simulink model "TWO_DOF_PID"  (R2023b)
settings: Solver=VariableStepAuto  StartTime=0.0  StopTime=10.0  RelTol=1e-3
undefined symbols (not defined in the file): beta_yaw, cneg, cpos, Dt, fd, force_coef, fs, I_omega, Jy, kTn1, kTn2, kTp1, kTp2, P_omega, parameters
libraries: slpidlib x3
settings Model: Creator=franc  LastModifiedBy=franc

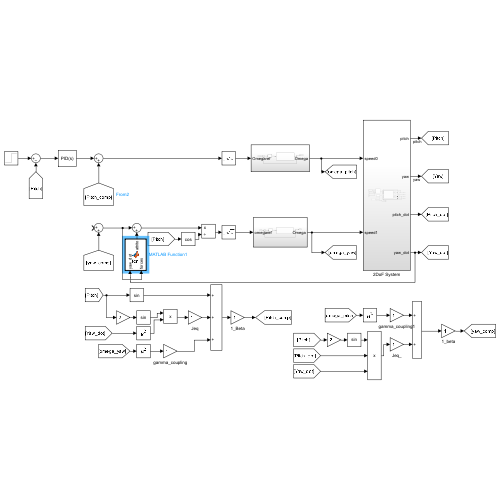
[thumbnail: Simulink's stored preview of the top-level diagram]
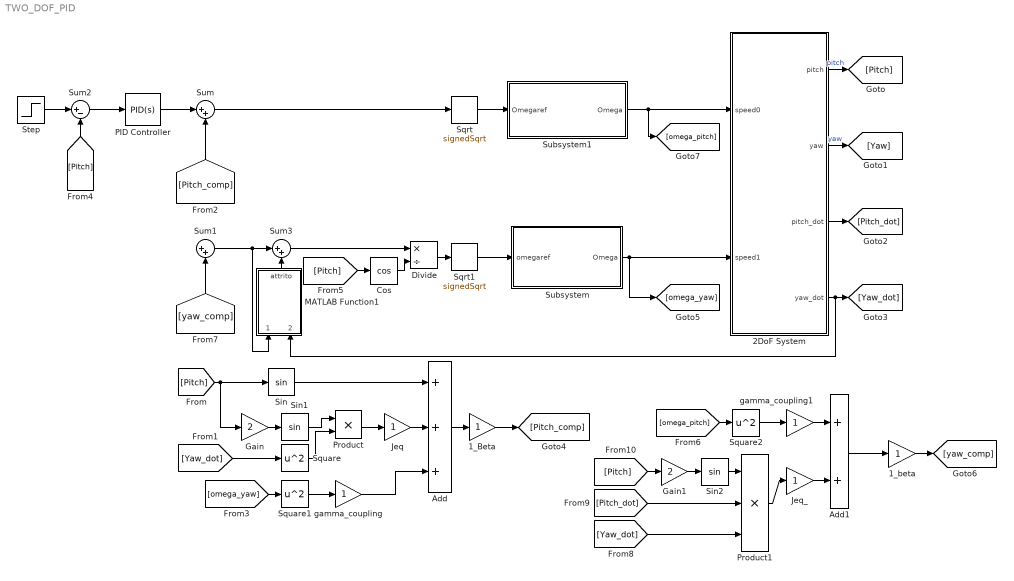
== system TWO_DOF_PID ==
  1_Beta : Gain
  1_beta : Gain
  2DoF System : Subsystem
  Add : Sum  Inputs=+++
  Add1 : Sum
  Cos : Trigonometry  Operator=cos
  Divide : Product  Inputs=*/
  Gain : Gain  Gain=2
  Gain1 : Gain  Gain=2
  Jeq : Gain
  Jeq_ : Gain
  MATLAB Function1 : MATLAB Function  TreatAsAtomicUnit=on
  PID Controller : slpidlib/PID Controller  Controller=PID  Form=Parallel  TimeDomain=Continuous-time  UseExternalTs=off  SampleTime=-1  IntegratorMethod=Forward Euler  FilterMethod=Forward Euler  ControllerParametersSource=internal  P=1  I=1  UseKiTs=off  D=0  N=100  UseFilter=on  TunerSelectOption=Transfer Function Based (PID Tuner App)  InitialConditionSource=internal  InitialConditionForIntegrator=0  InitialConditionForFilter=0  DifferentiatorICPrevScaledInput=0  ExternalReset=none  TrackingMode=off  Kt=1  LimitOutput=off  SatLimitsSource=internal  UpperSaturationLimit=inf  LowerSaturationLimit=-inf  LinearizeAsGain=on  AntiWindupMode=none  Kb=1  LimitIntegrator=off  UpperIntegratorSaturationLimit=inf  LowerIntegratorSaturationLimit=-inf  POutMin=[]  POutMax=[]  IOutMin=[]  IOutMax=[]  DOutMin=[]  DOutMax=[]  NOutMin=[]  NOutMax=[]  SumOutMin=[]  SumOutMax=[]  SaturationOutMin=[]  SaturationOutMax=[]  PParamMin=[]  PParamMax=[]  IParamMin=[]  IParamMax=[]  DParamMin=[]  DParamMax=[]  NParamMin=[]  NParamMax=[]  KbParamMin=[]  KbParamMax=[]  KtParamMin=[]  KtParamMax=[]  KbOutMin=[]  KbOutMax=[]  KtOutMin=[]  KtOutMax=[]  IntegratorOutMin=[]  IntegratorOutMax=[]  FilterOutMin=[]  FilterOutMax=[]  SumI1OutMin=[]  SumI1OutMax=[]  SumI2OutMin=[]  SumI2OutMax=[]  SumI3OutMin=[]  SumI3OutMax=[]  SumI4OutMin=[]  SumI4OutMax=[]  SumDOutMin=[]  SumDOutMax=[]  DifferentiatorOutMin=[]  DifferentiatorOutMax=[]  FilterDiffOutCoefMin=[]  FilterDiffOutCoefMax=[]  ReciprocalOutMin=[]  ReciprocalOutMax=[]  SumDenOutMin=[]  SumDenOutMax=[]  SumNumOutMin=[]  SumNumOutMax=[]  DivideOutMin=[]  DivideOutMax=[]  UdiffTsProdOutMin=[]  UdiffTsProdOutMax=[]  NTsProdOutMin=[]  NTsProdOutMax=[]  UintegralTsProdOutMin=[]  UintegralTsProdOutMax=[]  UngainTsProdOutMin=[]  UngainTsProdOutMax=[]  ClampingZeroOutDataTypeStr=Inherit: Inherit via back propagation  ClampingZeroOutMin=[]  ClampingZeroOutMax=[]  FilterDenConstantOutDataTypeStr=Inherit: Inherit via back propagation  FilterDenConstantOutMin=[]  FilterDenConstantOutMax=[]  PCopyOutDataTypeStr=Inherit: Inherit via back propagation  PCopyOutMin=[]  PCopyOutMax=[]  NCopyOutDataTypeStr=Inherit: Inherit via back propagation  NCopyOutMin=[]  NCopyOutMax=[]  IntegratorContinuousStateAttributes=''  IntegratorStateMustResolveToSignalObject=off  IntegratorRTWStateStorageClass=Auto  FilterContinuousStateAttributes=''  FilterStateMustResolveToSignalObject=off  FilterRTWStateStorageClass=Auto  ParallelPVariant=InternalParameters  IdealPVariant=Disabled  IVariant=InternalParameters  DVariant=InternalParameters  IntegratorVariant=Continuous  SatVariant=Disabled  AWVariant=Passthrough  PCopyVariant=Disabled  TRVariant=Disabled  FdbkBlocksVariant=Forward  IdealPFdbkVariant=Disabled  SatFdbkVariant=Disabled  DerivativeFilterVariant=ContFilter  NVariant=InternalParameters  NCopyVariant=Disabled  FilterICVariant=InternalICsFilter  IntegratorICVariant=InternalICs  ExternalResetVariant=Disabled  TRSumVariant=Passthrough  SumFdbkVariant=Disabled  SumVariant=Sum_PID  TsampFilterVariant=InternalTs  TsampNgainVariant=Passthrough  TsampIntegralVariant=Passthrough  ExternalSaturationOutDataTypeStr=Inherit: Same as second input
  Product : Product
  Product1 : Product  Inputs=3
  Sin : Trigonometry
  Sin1 : Trigonometry
  Sin2 : Trigonometry
  Sqrt : Sqrt  Operator=signedSqrt
  Sqrt1 : Sqrt  Operator=signedSqrt
  Square : Math  Operator=square
  Square1 : Math  Operator=square
  Square2 : Math  Operator=square
  Step : Step  After=30*pi/180  SampleTime=0
  Subsystem : Subsystem
  Subsystem1 : Subsystem
  Sum : Sum  Inputs=|++
  Sum1 : Sum  Inputs=|++
  Sum2 : Sum  Inputs=|+-
  Sum3 : Sum  Inputs=|++
  gamma_coupling : Gain
  gamma_coupling1 : Gain
  wires:
  Subsystem/1(Omega) -> [omega_yaw], 2DoF System/2(speed1)
  Subsystem1/1(Omega) -> [omega_pitch], 2DoF System/1(speed0)
  Sqrt/1 -> Subsystem1/1(Omegaref)
  Sqrt1/1 -> Subsystem/1(omegaref)
  Sum3/1 -> Divide/1
  Sum/1 -> Sqrt/1
  2DoF System/1(pitch) -> [Pitch]  "pitch"
  2DoF System/2(yaw) -> [Yaw]  "yaw"
  2DoF System/3(pitch_dot) -> [Pitch_dot]
  2DoF System/4(yaw_dot) -> MATLAB Function1/2(yaw_dot), [Yaw_dot]
  [Pitch] -> Gain/1, Sin/1
  Sin/1 -> Add/1
  Gain/1 -> Sin1/1
  Sin1/1 -> Product/1
  Jeq/1 -> Add/2
  [Yaw_dot] -> Square/1
  Product/1 -> Jeq/1
  Add/1 -> 1_Beta/1
  [Pitch_comp] -> Sum/2
  Square/1 -> Product/2
  [omega_yaw] -> Square1/1
  Square1/1 -> gamma_coupling/1
  gamma_coupling/1 -> Add/3
  PID Controller/1 -> Sum/1
  Sum2/1 -> PID Controller/1
  [Pitch] -> Sum2/2
  1_Beta/1 -> [Pitch_comp]
  Step/1 -> Sum2/1
  Divide/1 -> Sqrt1/1
  Cos/1 -> Divide/2
  [Pitch] -> Cos/1
  Add1/1 -> 1_beta/1
  1_beta/1 -> [yaw_comp]
  Square2/1 -> gamma_coupling1/1
  [omega_pitch] -> Square2/1
  gamma_coupling1/1 -> Add1/1
  [yaw_comp] -> Sum1/2
  Product1/1 -> Jeq_/1
  Jeq_/1 -> Add1/2
  [Yaw_dot] -> Product1/3
  [Pitch_dot] -> Product1/2
  Sin2/1 -> Product1/1
  Gain1/1 -> Sin2/1
  [Pitch] -> Gain1/1
  Sum1/1 -> MATLAB Function1/1(forces), Sum3/1
  MATLAB Function1/1(attrito) -> Sum3/2

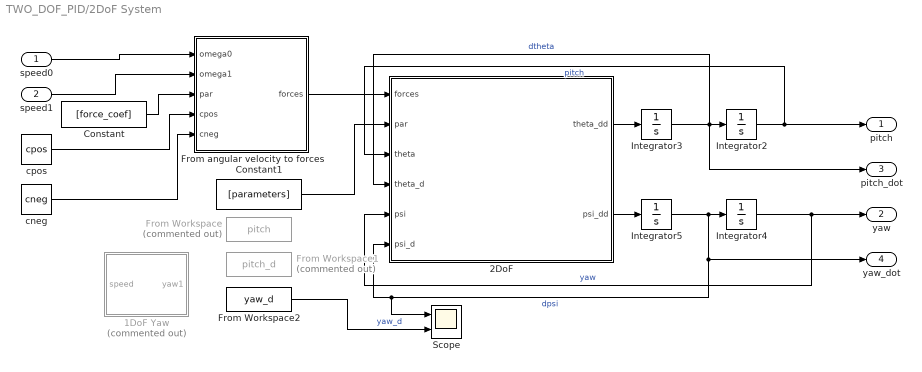
== system TWO_DOF_PID/2DoF System ==
  speed0 : Inport
  speed1 : Inport  Port=2
  1DoF Yaw : Subsystem  Commented=on
  2DoF : MATLAB Function  TreatAsAtomicUnit=on
  Constant : Constant  Value=[force_coef]
  Constant1 : Constant  Value=[parameters]
  From Workspace : FromWorkspace  Commented=on  VariableName=pitch  SampleTime=1/500
  From Workspace1 : FromWorkspace  Commented=on  VariableName=pitch_d  SampleTime=1/500
  From Workspace2 : FromWorkspace  VariableName=yaw_d  SampleTime=1/500
  From angular velocity to forces : MATLAB Function  TreatAsAtomicUnit=on
  Integrator{2..5} (4 alike) : Integrator
  Scope : Scope  NumInputPorts=2
  cneg : Constant  Value=cneg
  cpos : Constant  Value=cpos
  pitch : Outport
  yaw : Outport  Port=2
  pitch_dot : Outport  Port=3
  yaw_dot : Outport  Port=4
  wires:
  Integrator2/1 -> 2DoF/3(theta), pitch/1  "pitch"
  speed1/1 -> From angular velocity to forces/2(omega1)
  Integrator4/1 -> yaw/1, 2DoF/5(psi)  "yaw"
  speed0/1 -> From angular velocity to forces/1(omega0)
  2DoF/1(theta_dd) -> Integrator3/1
  From angular velocity to forces/1(forces) -> 2DoF/1(forces)
  Integrator3/1 -> pitch_dot/1, Integrator2/1, 2DoF/4(theta_d)  "dtheta"
  2DoF/2(psi_dd) -> Integrator5/1
  Integrator5/1 -> Integrator4/1, yaw_dot/1, Scope/1, 2DoF/6(psi_d)  "dpsi"
  Constant/1 -> From angular velocity to forces/3(par)
  Constant1/1 -> 2DoF/2(par)
  cpos/1 -> From angular velocity to forces/4(cpos)
  cneg/1 -> From angular velocity to forces/5(cneg)
  From Workspace2/1 -> Scope/2  "yaw_d"

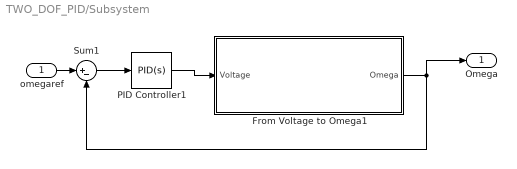
== system TWO_DOF_PID/Subsystem ==
  omegaref : Inport
  From Voltage to Omega1 : Subsystem
  PID Controller1 : slpidlib/PID Controller  Controller=PID  Form=Parallel  TimeDomain=Continuous-time  UseExternalTs=off  SampleTime=-1  IntegratorMethod=Forward Euler  FilterMethod=Forward Euler  ControllerParametersSource=internal  P=P_omega  I=I_omega  UseKiTs=off  D=0  N=100  UseFilter=on  TunerSelectOption=Transfer Function Based (PID Tuner App)  InitialConditionSource=internal  InitialConditionForIntegrator=0  InitialConditionForFilter=0  DifferentiatorICPrevScaledInput=0  ExternalReset=none  TrackingMode=off  Kt=1  LimitOutput=on  SatLimitsSource=internal  UpperSaturationLimit=18  LowerSaturationLimit=-18  LinearizeAsGain=on  AntiWindupMode=none  Kb=1  LimitIntegrator=off  UpperIntegratorSaturationLimit=inf  LowerIntegratorSaturationLimit=-inf  POutMin=[]  POutMax=[]  IOutMin=[]  IOutMax=[]  DOutMin=[]  DOutMax=[]  NOutMin=[]  NOutMax=[]  SumOutMin=[]  SumOutMax=[]  SaturationOutMin=[]  SaturationOutMax=[]  PParamMin=[]  PParamMax=[]  IParamMin=[]  IParamMax=[]  DParamMin=[]  DParamMax=[]  NParamMin=[]  NParamMax=[]  KbParamMin=[]  KbParamMax=[]  KtParamMin=[]  KtParamMax=[]  KbOutMin=[]  KbOutMax=[]  KtOutMin=[]  KtOutMax=[]  IntegratorOutMin=[]  IntegratorOutMax=[]  FilterOutMin=[]  FilterOutMax=[]  SumI1OutMin=[]  SumI1OutMax=[]  SumI2OutMin=[]  SumI2OutMax=[]  SumI3OutMin=[]  SumI3OutMax=[]  SumI4OutMin=[]  SumI4OutMax=[]  SumDOutMin=[]  SumDOutMax=[]  DifferentiatorOutMin=[]  DifferentiatorOutMax=[]  FilterDiffOutCoefMin=[]  FilterDiffOutCoefMax=[]  ReciprocalOutMin=[]  ReciprocalOutMax=[]  SumDenOutMin=[]  SumDenOutMax=[]  SumNumOutMin=[]  SumNumOutMax=[]  DivideOutMin=[]  DivideOutMax=[]  UdiffTsProdOutMin=[]  UdiffTsProdOutMax=[]  NTsProdOutMin=[]  NTsProdOutMax=[]  UintegralTsProdOutMin=[]  UintegralTsProdOutMax=[]  UngainTsProdOutMin=[]  UngainTsProdOutMax=[]  ClampingZeroOutDataTypeStr=Inherit: Inherit via back propagation  ClampingZeroOutMin=[]  ClampingZeroOutMax=[]  FilterDenConstantOutDataTypeStr=Inherit: Inherit via back propagation  FilterDenConstantOutMin=[]  FilterDenConstantOutMax=[]  PCopyOutDataTypeStr=Inherit: Inherit via back propagation  PCopyOutMin=[]  PCopyOutMax=[]  NCopyOutDataTypeStr=Inherit: Inherit via back propagation  NCopyOutMin=[]  NCopyOutMax=[]  IntegratorContinuousStateAttributes=''  IntegratorStateMustResolveToSignalObject=off  IntegratorRTWStateStorageClass=Auto  FilterContinuousStateAttributes=''  FilterStateMustResolveToSignalObject=off  FilterRTWStateStorageClass=Auto  ParallelPVariant=InternalParameters  IdealPVariant=Disabled  IVariant=InternalParameters  DVariant=InternalParameters  IntegratorVariant=Continuous  SatVariant=Enabled  AWVariant=Passthrough  PCopyVariant=Disabled  TRVariant=Disabled  FdbkBlocksVariant=Forward  IdealPFdbkVariant=Disabled  SatFdbkVariant=Disabled  DerivativeFilterVariant=ContFilter  NVariant=InternalParameters  NCopyVariant=Disabled  FilterICVariant=InternalICsFilter  IntegratorICVariant=InternalICs  ExternalResetVariant=Disabled  TRSumVariant=Passthrough  SumFdbkVariant=Disabled  SumVariant=Sum_PID  TsampFilterVariant=InternalTs  TsampNgainVariant=Passthrough  TsampIntegralVariant=Disabled_SignalSpec  ExternalSaturationOutDataTypeStr=Inherit: Same as second input
  Sum1 : Sum  Inputs=|+-
  Omega : Outport
  wires:
  From Voltage to Omega1/1(Omega) -> Omega/1, Sum1/2
  PID Controller1/1 -> From Voltage to Omega1/1(Voltage)
  Sum1/1 -> PID Controller1/1
  omegaref/1 -> Sum1/1

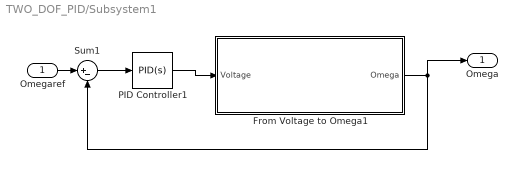
== system TWO_DOF_PID/Subsystem1 ==
  Omegaref : Inport
  From Voltage to Omega1 : Subsystem
  PID Controller1 : slpidlib/PID Controller  Controller=PID  Form=Parallel  TimeDomain=Continuous-time  UseExternalTs=off  SampleTime=-1  IntegratorMethod=Forward Euler  FilterMethod=Forward Euler  ControllerParametersSource=internal  P=P_omega  I=I_omega  UseKiTs=off  D=0  N=100  UseFilter=on  TunerSelectOption=Transfer Function Based (PID Tuner App)  InitialConditionSource=internal  InitialConditionForIntegrator=0  InitialConditionForFilter=0  DifferentiatorICPrevScaledInput=0  ExternalReset=none  TrackingMode=off  Kt=1  LimitOutput=on  SatLimitsSource=internal  UpperSaturationLimit=18  LowerSaturationLimit=-18  LinearizeAsGain=on  AntiWindupMode=none  Kb=1  LimitIntegrator=off  UpperIntegratorSaturationLimit=inf  LowerIntegratorSaturationLimit=-inf  POutMin=[]  POutMax=[]  IOutMin=[]  IOutMax=[]  DOutMin=[]  DOutMax=[]  NOutMin=[]  NOutMax=[]  SumOutMin=[]  SumOutMax=[]  SaturationOutMin=[]  SaturationOutMax=[]  PParamMin=[]  PParamMax=[]  IParamMin=[]  IParamMax=[]  DParamMin=[]  DParamMax=[]  NParamMin=[]  NParamMax=[]  KbParamMin=[]  KbParamMax=[]  KtParamMin=[]  KtParamMax=[]  KbOutMin=[]  KbOutMax=[]  KtOutMin=[]  KtOutMax=[]  IntegratorOutMin=[]  IntegratorOutMax=[]  FilterOutMin=[]  FilterOutMax=[]  SumI1OutMin=[]  SumI1OutMax=[]  SumI2OutMin=[]  SumI2OutMax=[]  SumI3OutMin=[]  SumI3OutMax=[]  SumI4OutMin=[]  SumI4OutMax=[]  SumDOutMin=[]  SumDOutMax=[]  DifferentiatorOutMin=[]  DifferentiatorOutMax=[]  FilterDiffOutCoefMin=[]  FilterDiffOutCoefMax=[]  ReciprocalOutMin=[]  ReciprocalOutMax=[]  SumDenOutMin=[]  SumDenOutMax=[]  SumNumOutMin=[]  SumNumOutMax=[]  DivideOutMin=[]  DivideOutMax=[]  UdiffTsProdOutMin=[]  UdiffTsProdOutMax=[]  NTsProdOutMin=[]  NTsProdOutMax=[]  UintegralTsProdOutMin=[]  UintegralTsProdOutMax=[]  UngainTsProdOutMin=[]  UngainTsProdOutMax=[]  ClampingZeroOutDataTypeStr=Inherit: Inherit via back propagation  ClampingZeroOutMin=[]  ClampingZeroOutMax=[]  FilterDenConstantOutDataTypeStr=Inherit: Inherit via back propagation  FilterDenConstantOutMin=[]  FilterDenConstantOutMax=[]  PCopyOutDataTypeStr=Inherit: Inherit via back propagation  PCopyOutMin=[]  PCopyOutMax=[]  NCopyOutDataTypeStr=Inherit: Inherit via back propagation  NCopyOutMin=[]  NCopyOutMax=[]  IntegratorContinuousStateAttributes=''  IntegratorStateMustResolveToSignalObject=off  IntegratorRTWStateStorageClass=Auto  FilterContinuousStateAttributes=''  FilterStateMustResolveToSignalObject=off  FilterRTWStateStorageClass=Auto  ParallelPVariant=InternalParameters  IdealPVariant=Disabled  IVariant=InternalParameters  DVariant=InternalParameters  IntegratorVariant=Continuous  SatVariant=Enabled  AWVariant=Passthrough  PCopyVariant=Disabled  TRVariant=Disabled  FdbkBlocksVariant=Forward  IdealPFdbkVariant=Disabled  SatFdbkVariant=Disabled  DerivativeFilterVariant=ContFilter  NVariant=InternalParameters  NCopyVariant=Disabled  FilterICVariant=InternalICsFilter  IntegratorICVariant=InternalICs  ExternalResetVariant=Disabled  TRSumVariant=Passthrough  SumFdbkVariant=Disabled  SumVariant=Sum_PID  TsampFilterVariant=InternalTs  TsampNgainVariant=Passthrough  TsampIntegralVariant=Disabled_SignalSpec  ExternalSaturationOutDataTypeStr=Inherit: Same as second input
  Sum1 : Sum  Inputs=|+-
  Omega : Outport
  wires:
  From Voltage to Omega1/1(Omega) -> Omega/1, Sum1/2
  PID Controller1/1 -> From Voltage to Omega1/1(Voltage)
  Sum1/1 -> PID Controller1/1
  Omegaref/1 -> Sum1/1

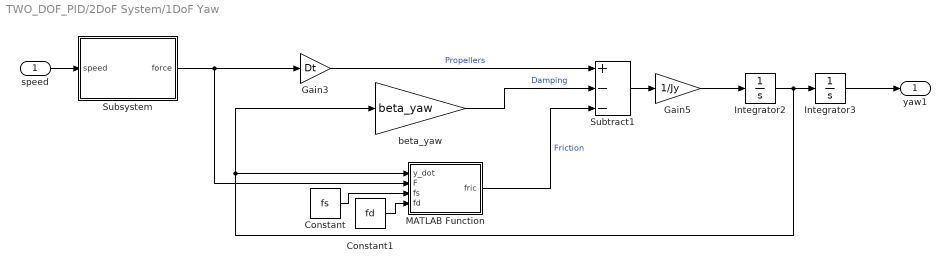
== system TWO_DOF_PID/2DoF System/1DoF Yaw ==
  speed : Inport
  Constant : Constant  Value=fs
  Constant1 : Constant  Value=fd
  Gain3 : Gain  Gain=Dt
  Gain5 : Gain  Gain=1/Jy
  Integrator2 : Integrator
  Integrator3 : Integrator
  MATLAB Function : MATLAB Function  TreatAsAtomicUnit=on
  Subsystem : Subsystem
  Subtract1 : Sum  Inputs=+--
  beta_yaw : Gain  Gain=beta_yaw
  yaw1 : Outport
  wires:
  Integrator3/1 -> yaw1/1
  Subtract1/1 -> Gain5/1
  Gain5/1 -> Integrator2/1
  Integrator2/1 -> Integrator3/1, beta_yaw/1, MATLAB Function/1(y_dot)
  MATLAB Function/1(fric) -> Subtract1/3  "Friction"
  beta_yaw/1 -> Subtract1/2  "Damping"
  Gain3/1 -> Subtract1/1  "Propellers"
  Constant/1 -> MATLAB Function/3(fs)
  Constant1/1 -> MATLAB Function/4(fd)
  Subsystem/1(force) -> Gain3/1, MATLAB Function/2(F)
  speed/1 -> Subsystem/1(speed)

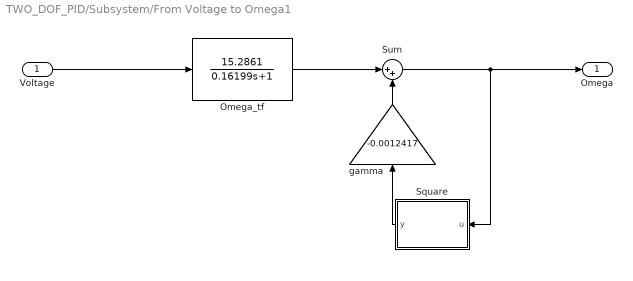
== system TWO_DOF_PID/Subsystem/From Voltage to Omega1 ==
  Voltage : Inport
  Omega_tf : TransferFcn  Numerator=15.2861  Denominator=[0.16199 1]
  Square : MATLAB Function  TreatAsAtomicUnit=on
  Sum : Sum  Inputs=|++
  gamma : Gain  Gain=-0.0012417
  Omega : Outport
  wires:
  Voltage/1 -> Omega_tf/1
  gamma/1 -> Sum/2
  Square/1(y) -> gamma/1
  Omega_tf/1 -> Sum/1
  Sum/1 -> Omega/1, Square/1(u)

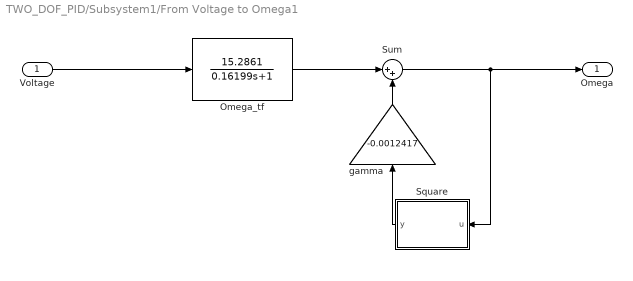
== system TWO_DOF_PID/Subsystem1/From Voltage to Omega1 ==
  Voltage : Inport
  Omega_tf : TransferFcn  Numerator=15.2861  Denominator=[0.16199 1]
  Square : MATLAB Function  TreatAsAtomicUnit=on
  Sum : Sum  Inputs=|++
  gamma : Gain  Gain=-0.0012417
  Omega : Outport
  wires:
  Voltage/1 -> Omega_tf/1
  gamma/1 -> Sum/2
  Square/1(y) -> gamma/1
  Omega_tf/1 -> Sum/1
  Sum/1 -> Omega/1, Square/1(u)

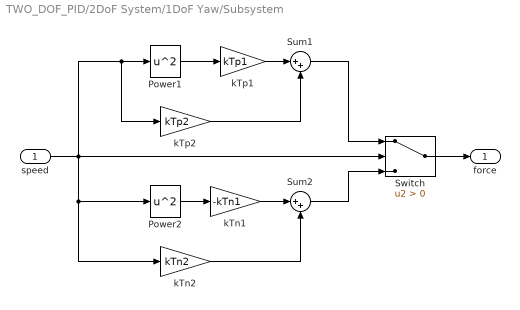
== system TWO_DOF_PID/2DoF System/1DoF Yaw/Subsystem ==
  speed : Inport
  Power1 : Math  Operator=square  SignedPower=on
  Power2 : Math  Operator=square  SignedPower=on
  Sum1 : Sum  Inputs=|++
  Sum2 : Sum  Inputs=|++
  Switch : Switch  Criteria=u2 > Threshold  SaturateOnIntegerOverflow=off  InputSameDT=off
  kTn1 : Gain  Gain=-kTn1
  kTn2 : Gain  Gain=kTn2
  kTp1 : Gain  Gain=kTp1
  kTp2 : Gain  Gain=kTp2
  force : Outport
  wires:
  kTp1/1 -> Sum1/1
  speed/1 -> Switch/2, kTn2/1, Power2/1, Power1/1, kTp2/1
  kTn2/1 -> Sum2/2
  Power2/1 -> kTn1/1
  Sum2/1 -> Switch/3
  Power1/1 -> kTp1/1
  kTn1/1 -> Sum2/1
  kTp2/1 -> Sum1/2
  Sum1/1 -> Switch/1
  Switch/1 -> force/1

== matlab function TWO_DOF_PID/2DoF System/1DoF Yaw/MATLAB Function ==
  data: y_dot input; fric output; F input; fs input; fd input
function fric = fcn(y_dot, F, fs, fd)

fric  = abs(F);
if fric > fs || y_dot ~= 0
    fric = fd;
end

fric = fric*sign(y_dot);

== matlab function TWO_DOF_PID/2DoF System/2DoF ==
  data: forces input; par input; theta input; theta_d input; psi input; psi_d input; theta_dd output; psi_dd output
function [theta_dd, psi_dd]  = model_2dof(forces, par, theta, theta_d, psi, psi_d)%, real_pitch, real_pitch_d, real_yaw_d)

% Assumed to be known parameters
Mb = 1.07; % mass of the upper body
d = 0.0024; % missalignment of the c.o.m. of the upper body
Dt = 0.167; % distance between yaw axis of rotation to motor axis
g = 9.81;

%used in Pitch EoM
yaw_d = psi_d;
% yaw_d = real_yaw_d;

% used in Yaw EoM
pitch = theta;
pitch_d = theta_d;
% pitch = real_pitch;
% pitch_d = real_pitch_d;

% Forces applied 
F0 = forces(1);
F1 = forces(2);
Q0 = forces(3);
Q1 = forces(4);

% Inertia of lower body w.r.t. its local reference frame.
Jx1 = par(1);
Jy1 = par(2);
Jz1 = par(3);

% Inertial of upper body w.r.t its local reference frame.
Jx2 = par(4);
Jy2 = par(5);
Jz2 = par(6);

beta_pitch = par(7); % Damping due to yaw rotation
beta_yaw = par(8); % Damping due to pitch rotation

fs = par(9);
fd = par(10);

mode = par(11);

% Coefficents multiplied by theta_dot_dot
J_theta = Jy2 + Mb*d^2;
% Coefficents multiplied by psi_dot_dot
J_psi = Jz1 + Jx2*sin(pitch)^2 + Jz2*cos(pitch)^2 + Mb*d^2*sin(pitch)^2;
% J_psi = Jz1+Jz2; % for 1 DoF Yaw

switch mode
    case 0
        tau_pitch = (F0-F1)*Dt;
        tau_yaw = 0;
    case 1
        tau_pitch = 0;
        tau_yaw = (F0+F1)*Dt*cos(pitch);
    otherwise
        tau_pitch = F0*Dt-Q1;
        % tau_pitch = F0*Dt; % for 1 DoF Pitch
        tau_yaw = (F1*Dt+Q0)*cos(pitch);
        % tau_yaw = (F1*Dt); % for 1 DoF Yaw
end

% Yaw Friction
fric  = abs(tau_yaw);
if fric > fs || abs(psi_d) > 1
    fric = fd;
end
fric = fric*sign(psi_d); % as the friction force is always oppostite to the movement

coupling_term_pitch = -0.5*(Jx2-Jz2+Mb*d^2)*sin(2*theta)*yaw_d^2;
% coupling_term_pitch = 0; % for 1 DoF Pitch
theta_dd = (tau_pitch - beta_pitch*theta_d - coupling_term_pitch - Mb*g*d*sin(theta))/J_theta;

coupling_term_yaw = (Jx2-Jz2+Mb*d^2)*sin(2*pitch)*psi_d*pitch_d;
% coupling_term_yaw = 0; % for 1 DoF Yaw
psi_dd = (tau_yaw - beta_yaw*psi_d - coupling_term_yaw - fric)/J_psi;

== matlab function TWO_DOF_PID/2DoF System/From angular velocity to forces ==
  data: omega0 input; forces output; omega1 input; par input; cpos input; cneg input
function forces = fcn(omega0, omega1, par, cpos, cneg)

kTp1 = par(1);
kTp2 = par(2);

kTn1 = par(3);
kTn2 = par(4);

cQ0 = cpos;
cQ1 = cpos;

cQ0n = cneg;
cQ1n = cneg;

if omega0 > 0
    F0 = kTp1*omega0^2 + kTp2*omega0;
    Q0 = 1.5*cQ0*omega0^2;
else
    F0 = (-kTn1*omega0^2 + kTn2*omega0);
    Q0 = -0.5*cQ0n*omega0^2;
end

if omega1 > 0
    F1 = kTp1*omega1^2 + kTp2*omega1;
    Q1 = cQ1*omega1^2;
else
    F1 = 0.05*(-kTn1*omega1^2 + kTn2*omega1);
    Q1 = -0.5*cQ1n*omega1^2;
end

forces = [F0,F1,Q0,Q1];

end

== matlab function TWO_DOF_PID/Subsystem1/From Voltage to Omega1/Square ==
  data: u input; y output
function y = fcn(u)
y=u^2*sign(u);

== matlab function TWO_DOF_PID/Subsystem/From Voltage to Omega1/Square ==
  data: u input; y output
function y = fcn(u)
y=u^2*sign(u);

== matlab function TWO_DOF_PID/MATLAB Function1 ==
  data: forces input; yaw_dot input; attrito output
function attrito = fcn(forces,yaw_dot)
fd=0.0035;
fs=0.0088;

attrito=abs(forces);

if attrito>fs || abs(yaw_dot)>=1
    attrito=fd;
end

attrito=attrito*sign(yaw_dot);
